simulink model "ES249A_MotAgCorrln"  (R2013b)
settings: Solver=FixedStepDiscrete  SolverMode=SingleTasking  StartTime=0.0  StopTime=1  FixedStep=0.002  RelTol=1e-3
undefined symbols (not defined in the file): FLTINJ_MOTAGCORRLN_MOTAGIDPTSIG, HALFREV_MOTREV_U0P16, MOTAGACORRLNST_CNT_U08, MotAgAMotAgBCorrln, MotAgAMotAgCCorrln, MOTAGBCORRLNST_CNT_U08, MotAgBMotAgCCorrln, MOTAGCCORRLNST_CNT_U08, MOTAGCORRLNERRTHD_MOTREVELEC_U0P16, MOTAGCORRLNNTCFAILSTEP_CNT_U16, MOTAGCORRLNNTCPASSSTEP_CNT_U16, MOTAGMAXSTALLCNTR_CNT_U08, MotAgMeclCorrlnSt, MotAgMeclIdptSig, NtcSts1, sigbuilder_block, SysGlbPrmMotPoleCnt
libraries: simulink x5
(part 1 of 4)
settings Model: Creator=pz79n7  LastModifiedBy=FZG88Y
settings SolverCC: AutoInsertRateTranBlk=on  InsertRTBMode=Always
settings DataIOCC: LimitDataPoints=off  SaveFormat=Structure  ReturnWorkspaceOutputs=on
settings OptimizationCC: BlockReduction=off  InlineParams=on  ZeroExternalMemoryAtStartup=off  ZeroInternalMemoryAtStartup=off  OptimizeModelRefInitCode=on  LifeSpan=1
settings DebuggingCC: SignalInfNanChecking=error  SignalRangeChecking=warning  UnderspecifiedInitializationDetection=Simplified  SolverPrmCheckMsg=error  InheritedTsInSrcMsg=error  DiscreteInheritContinuousMsg=error  SingleTaskRateTransMsg=error  TasksWithSamePriorityMsg=error  SigSpecEnsureSampleTimeMsg=error  CheckMatrixSingularityMsg=error  ParameterUnderflowMsg=error  ParameterPrecisionLossMsg=error  ParameterTunabilityLossMsg=error  FixptConstUnderflowMsg=warning  FixptConstOverflowMsg=warning  VectorMatrixConversionMsg=error  SignalLabelMismatchMsg=error  UnconnectedInputMsg=error  UnconnectedOutputMsg=error  UnconnectedLineMsg=error  SFcnCompatibilityMsg=error  UniqueDataStoreMsg=warning  BusObjectLabelMismatch=error  RootOutportRequireBusObject=error  AssertControl=DisableAll  ModelReferenceIOMsg=error  ModelReferenceVersionMismatchMessage=warning  ModelReferenceIOMismatchMessage=error  ModelReferenceCSMismatchMessage=warning  ModelReferenceDataLoggingMessage=error  StateNameClashWarn=warning  StrictBusMsg=ErrorOnBusTreatedAsVector  NonBusSignalsTreatedAsBus=error  SFUnexpectedBacktrackingDiag=error  SFInvalidInputDataAccessInChartInitDiag=error  SFNoUnconditionalDefaultTransitionDiag=error  SFTransitionOutsideNaturalParentDiag=error  SFUnconditionalTransitionShadowingDiag=error  SFUndirectedBroadcastEventsDiag=error
settings ModelReferenceCC: ModelReferenceNumInstancesAllowed=Single
settings RTWCC: SystemTargetFile=autosar.tlc  GenCodeOnly=on  TemplateMakefile=ert_default_tmf  Description=AUTOSAR  GenerateReport=on  ProcessScript=autosar_make_rtw_hook  LaunchReport=on
settings CodeAppCC: GenerateComments=off  IgnoreCustomStorageClasses=off  CustomSymbolStrType=$N$R$M  CustomSymbolStrBlkIO=$N$M  SimulinkBlockComments=off
settings STFCustomTargetCC: ParMdlRefBuildCompliant=on  CompOptLevelCompliant=on  IncludeMdlTerminateFcn=off  CombineOutputUpdateFcns=on  SuppressErrorStatus=on  ERTFirstTimeCompliant=on  ERTCustomFileBanners=on  SupportNonFinite=off  SupportComplex=off  SupportContinuousTime=off  SupportNonInlinedSFcns=off  MATLABClassNameForMDSCustomization=Simulink.SoftwareTarget.ERTCustomization  AutosarCompliant=on  GRTInterface=off  SystemTargetFile=autosar.tlc
settings ERTTargetCC: CodeReplacementLibrary=ANSI_C  ConcurrentExecutionCompliant=off  IncludeMdlTerminateFcn=off  SuppressErrorStatus=on  SupportNonFinite=off  SupportComplex=off  ModelStepFunctionPrototypeControlCompliant=off  CPPClassGenCompliant=off  AutosarCompliant=on  InlinedParameterPlacement=NonHierarchical  ERTCustomFileTemplate=example_file_process.tlc  EnableUserReplacementTypes=on

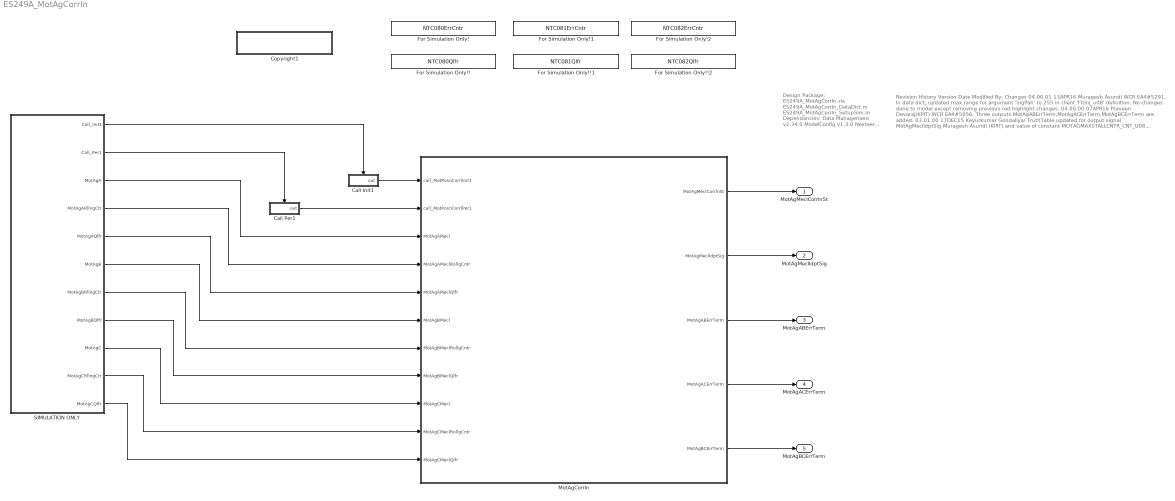
== system ES249A_MotAgCorrln ==
  note: Revision History
      |
      | Version		Date 		Modified By: 		          Changes
      | 04.00.01        13APR16     Muragesh Asundi              WCR EA4#5291, In data dict, updated max range for argument 'SigPah' to 255 in client 'FltInj_u08' definition.
      |                                                                                     No changes done to model except removing previous red highlight changes.
      | 04.00.00        07APR16      Praveen Devaraj(KPIT)    WCR EA4#5056. Three outputs MotAgABErrTerm,MotAgACErrTerm,MotAgBCErrTerm are added.
      | 03.01.00        17DEC15      Keyurkumar Gondaliya/    TruthTable updated for output signal MotAgMeclIdptSig
      |                                             Muragesh Asundi (KPIT)  and value of constant MOTAGMAXSTALLCNTR_CNT_U08
      |                                                                                      changed to 200. Work CR EA4#2808
      | 03.00.00		12NOV15	Erlenbeck		            EA4#2424 anomaly cleanup.  Need to account
      | 										            for rollover in correlation diagnostic.
      | 02.01.01        24AUG15      Muragesh Asundi             Data Dict updated for FltInj_u08 arg2 data type
      |                                                                                      per CR EA4#1391
      | 02.01.00        20AUG15      Muragesh Asundi             Rename FltInj & Bit Set/Not Set Anomaly
      |  										           per CR EA4#1353
      | 02.00.00        07AUG15      Aditya Tikekar                  Fault Injection added for MotAgMeclIdptSig
      |  										           per CR EA4#1161
      | 01.00.00 	02AP15		Kushion			            Initial Release
  note: Design Package:
      | ES249A_MotAgCorrln.slx
      | ES249A_MotAgCorrln_DataDict.m
      | ES249A_MotAgCorrln_SetupSim.m
      |
      | Dependancies:
      |    Data Management v2.34.0
      |    ModelConfig v1.3.0
      |    Nexteer Utilities v4.5.0
      |    Tools v1.10.0
      |
      | Requirement: 2.0
  Call Init1 : Subsystem  TreatAsAtomicUnit=on
  Call Per1 : Subsystem  TreatAsAtomicUnit=on
  Copyright1 : Subsystem  Description=|  mask(Copyright Information){none=on}
      | Copyright info block.                                               
      |                                                                     
      | Place copyright information at the top of every subsystem in design.
      mask prompts: none "No parameters"
      mask help: Place copyright information at the top of every subsystem in design.
      mask Display:
      | NxtrConf = 'Nexteer Confidential';
      | 
      | sys = bdroot; %handle for the current model ("system")
      | first = get_param(sys,'Created');
      | if(isempty(first))
      |     first = datestr(now,'yyyy');
      | else
      |     first = first(end-3:end);  %year is last four digits
      | end
      | 
      | last = get_param(sys,'LastModifiedDate');
      | if isempty(last)
      |     last = datestr(now,'yyyy');
      | else
      |     last = last(end-3:end);
      | end
      | 
      | if strcmp(first,last)
      |     fprintf('%s\nCopyright  %s Nexteer',NxtrConf,first);
      | else
      |     fprintf('%s\n%s%s-%s Nexteer',NxtrConf,char(169),first,last);
      | end
  For Simulation Only! : DataStoreMemory  DataStoreName=NTC080ErrCntr
  For Simulation Only!! : DataStoreMemory  DataStoreName=NTC080Qlfr
  For Simulation Only!!1 : DataStoreMemory  DataStoreName=NTC081Qlfr
  For Simulation Only!!2 : DataStoreMemory  DataStoreName=NTC082Qlfr
  For Simulation Only!1 : DataStoreMemory  DataStoreName=NTC081ErrCntr
  For Simulation Only!2 : DataStoreMemory  DataStoreName=NTC082ErrCntr
  MotAgCorrln : Subsystem
  SIMULATION ONLY : Subsystem
  MotAgMeclCorrlnSt : Outport  RequirementInfo={'linktype_rmi_doors' '0000c47a (/E-STEER Core/SubSystem Specifications/Electrical Actuator/Control Module/FDD Module Requirements/EA4/ES249A_MotAgCorrln DRAFT)' '#ES249A_51' 'true' 'REQ: ES249A_51' '' } %GIDa_d8739ec6_a18f_4415_a443_47ea44f287a3
  MotAgMeclIdptSig : Outport  RequirementInfo={'linktype_rmi_doors' '0000c47a (/E-STEER Core/SubSystem Specifications/Electrical Actuator/Control Module/FDD Module Requirements/EA4/ES249A_MotAgCorrln DRAFT)' '#ES249A_52' 'true' 'REQ: ES249A_52' '' } %GIDa_85b325d8_f6bf_41e3_b16b_50e782c8add7  Port=2
  MotAgABErrTerm : Outport  Port=3
  MotAgACErrTerm : Outport  Port=4
  MotAgBCErrTerm : Outport  Port=5
  wires:
  Call Per1/1(out) -> MotAgCorrln/2(call_MotPosnCorrlPer1)
  MotAgCorrln/1(MotAgMeclCorrlnSt) -> MotAgMeclCorrlnSt/1
  MotAgCorrln/2(MotAgMeclIdptSig) -> MotAgMeclIdptSig/1
  SIMULATION ONLY/3(MotAgA) -> MotAgCorrln/3(MotAgAMecl)
  SIMULATION ONLY/11(MotAgCQlfr) -> MotAgCorrln/11(MotAgCMeclQlfr)
  SIMULATION ONLY/4(MotAgARllngCtr) -> MotAgCorrln/4(MotAgAMeclRollgCntr)
  SIMULATION ONLY/5(MotAgAQlfr) -> MotAgCorrln/5(MotAgAMeclQlfr)
  SIMULATION ONLY/6(MotAgB) -> MotAgCorrln/6(MotAgBMecl)
  SIMULATION ONLY/7(MotAgBRllngCtr) -> MotAgCorrln/7(MotAgBMeclRollgCntr)
  SIMULATION ONLY/8(MotAgBQlfr) -> MotAgCorrln/8(MotAgBMeclQlfr)
  SIMULATION ONLY/9(MotAgC) -> MotAgCorrln/9(MotAgCMecl)
  SIMULATION ONLY/10(MotAgCRllngCtr) -> MotAgCorrln/10(MotAgCMeclRollgCntr)
  Call Init1/1(out) -> MotAgCorrln/1(call_MotPosnCorrlInit1)
  SIMULATION ONLY/1(Call_Init1) -> Call Init1/Enable
  SIMULATION ONLY/2(Call_Per1) -> Call Per1/Enable
  MotAgCorrln/3(MotAgABErrTerm) -> MotAgABErrTerm/1
  MotAgCorrln/4(MotAgACErrTerm) -> MotAgACErrTerm/1
  MotAgCorrln/5(MotAgBCErrTerm) -> MotAgBCErrTerm/1

== system ES249A_MotAgCorrln/Call Init1 ==
  Enable : EnablePort
  Function Call Trigger : simulink/Ports & Subsystems/Function-Call Generator  RequirementInfo={} %GIDa_ff755a2e_49d1_45f7_8591_3ce0ef475338  sample_time=0  numberOfIterations=1
  out : Outport
  wires:
  Function Call Trigger/1 -> out/1

== system ES249A_MotAgCorrln/Call Per1 ==
  Enable : EnablePort
  Function Call Trigger : simulink/Ports & Subsystems/Function-Call Generator  RequirementInfo={} %GIDa_c055ea22_668e_465c_aa17_4b0a8dd99bf7  sample_time=0.002  numberOfIterations=1
  out : Outport
  wires:
  Function Call Trigger/1 -> out/1

== system ES249A_MotAgCorrln/Copyright1 ==

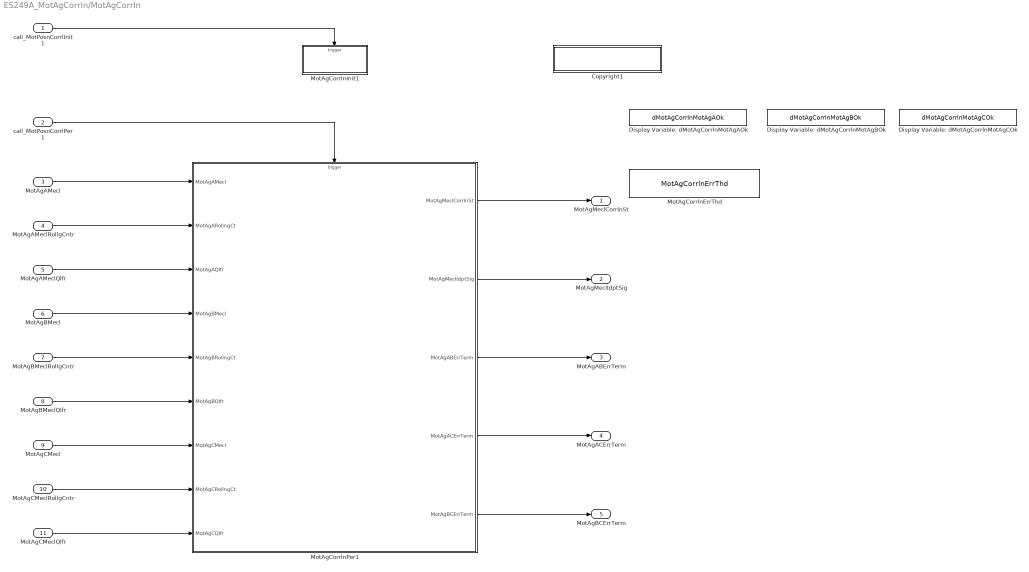
== system ES249A_MotAgCorrln/MotAgCorrln ==
  call_MotPosnCorrlInit1 : Inport  RequirementInfo={} %GIDa_df7b2033_8a98_4878_957d_25acf0131f4b
  call_MotPosnCorrlPer1 : Inport  RequirementInfo={} %GIDa_1551d67e_f818_426a_9cf4_9f4ba82b3f43  Port=2
  MotAgAMecl : Inport  RequirementInfo={'linktype_rmi_doors' '0000c47a (/E-STEER Core/SubSystem Specifications/Electrical Actuator/Control Module/FDD Module Requirements/EA4/ES249A_MotAgCorrln DRAFT)' '#ES249A_48' 'true' 'REQ: ES249A_48' '' } %GIDa_ab802314_3944_43a8_9f34_099947b7f787  Port=3
  MotAgAMeclRollgCntr : Inport  RequirementInfo={'linktype_rmi_doors' '0000c47a (/E-STEER Core/SubSystem Specifications/Electrical Actuator/Control Module/FDD Module Requirements/EA4/ES249A_MotAgCorrln DRAFT)' '#ES249A_49' 'true' 'REQ: ES249A_49' '' } %GIDa_a38bab73_f7bf_4755_8745_3afc46561306  Port=4
  MotAgAMeclQlfr : Inport  RequirementInfo={'linktype_rmi_doors' '0000c47a (/E-STEER Core/SubSystem Specifications/Electrical Actuator/Control Module/FDD Module Requirements/EA4/ES249A_MotAgCorrln DRAFT)' '#ES249A_65' 'true' 'REQ: ES249A_65' '' } %GIDa_033694cf_56a5_4107_96d0_836401cb9721  Port=5
  MotAgBMecl : Inport  RequirementInfo={'linktype_rmi_doors' '0000c47a (/E-STEER Core/SubSystem Specifications/Electrical Actuator/Control Module/FDD Module Requirements/EA4/ES249A_MotAgCorrln DRAFT)' '#ES249A_66' 'true' 'REQ: ES249A_66' '' } %GIDa_ed21c9ba_4edb_4b2f_a77a_49cd20ecbf68  Port=6
  MotAgBMeclRollgCntr : Inport  RequirementInfo={'linktype_rmi_doors' '0000c47a (/E-STEER Core/SubSystem Specifications/Electrical Actuator/Control Module/FDD Module Requirements/EA4/ES249A_MotAgCorrln DRAFT)' '#ES249A_67' 'true' 'REQ: ES249A_67' '' } %GIDa_6e6bb4b4_2d5c_4f1b_b4e7_5884c06a9259  Port=7
  MotAgBMeclQlfr : Inport  RequirementInfo={'linktype_rmi_doors' '0000c47a (/E-STEER Core/SubSystem Specifications/Electrical Actuator/Control Module/FDD Module Requirements/EA4/ES249A_MotAgCorrln DRAFT)' '#ES249A_68' 'true' 'REQ: ES249A_68' '' } %GIDa_842dc15f_0b28_4c0e_80ed_768af48a7cab  Port=8
  MotAgCMecl : Inport  RequirementInfo={'linktype_rmi_doors' '0000c47a (/E-STEER Core/SubSystem Specifications/Electrical Actuator/Control Module/FDD Module Requirements/EA4/ES249A_MotAgCorrln DRAFT)' '#ES249A_69' 'true' 'REQ: ES249A_69' '' } %GIDa_4e69db8b_365e_45b9_94df_b7de55be4fe5  Port=9
  MotAgCMeclRollgCntr : Inport  RequirementInfo={'linktype_rmi_doors' '0000c47a (/E-STEER Core/SubSystem Specifications/Electrical Actuator/Control Module/FDD Module Requirements/EA4/ES249A_MotAgCorrln DRAFT)' '#ES249A_70' 'true' 'REQ: ES249A_70' '' } %GIDa_8619747b_ec91_49fd_b968_535920207abf  Port=10
  MotAgCMeclQlfr : Inport  RequirementInfo={'linktype_rmi_doors' '0000c47a (/E-STEER Core/SubSystem Specifications/Electrical Actuator/Control Module/FDD Module Requirements/EA4/ES249A_MotAgCorrln DRAFT)' '#ES249A_71' 'true' 'REQ: ES249A_71' '' } %GIDa_ccdead46_e253_49ae_a139_b28c04022f0c  Port=11
  Copyright1 : Subsystem  Description=|  RequirementInfo={} %GIDa_dd7bc4e6_4adb_4397_9a47_107977c533a5  mask(Copyright Information){none=on}
      | Copyright info block.                                               
      |                                                                     
      | Place copyright information at the top of every subsystem in design.
      mask prompts: none "No parameters"
      mask help: Place copyright information at the top of every subsystem in design.
      mask Display:
      | NxtrConf = 'Nexteer Confidential';
      | 
      | sys = bdroot; %handle for the current model ("system")
      | first = get_param(sys,'Created');
      | if(isempty(first))
      |     first = datestr(now,'yyyy');
      | else
      |     first = first(end-3:end);  %year is last four digits
      | end
      | 
      | last = get_param(sys,'LastModifiedDate');
      | if isempty(last)
      |     last = datestr(now,'yyyy');
      | else
      |     last = last(end-3:end);
      | end
      | 
      | if strcmp(first,last)
      |     fprintf('%s\nCopyright  %s Nexteer',NxtrConf,first);
      | else
      |     fprintf('%s\n%s%s-%s Nexteer',NxtrConf,char(169),first,last);
      | end
  Display Variable: dMotAgCorrlnMotAgAOk : DataStoreMemory  DataStoreName=dMotAgCorrlnMotAgAOk  StateMustResolveToSignalObject=on
  Display Variable: dMotAgCorrlnMotAgBOk : DataStoreMemory  DataStoreName=dMotAgCorrlnMotAgBOk  StateMustResolveToSignalObject=on
  Display Variable: dMotAgCorrlnMotAgCOk : DataStoreMemory  DataStoreName=dMotAgCorrlnMotAgCOk  StateMustResolveToSignalObject=on
  MotAgCorrlnErrThd : DataStoreMemory  Priority=0  DataStoreName=MotAgCorrlnErrThd  StateMustResolveToSignalObject=on
  MotAgCorrlnInit1 : Subsystem  TreatAsAtomicUnit=on
  MotAgCorrlnPer1 : Subsystem  RequirementInfo={} %GIDa_e8c7526b_9849_4008_8b1a_56f97ffa1c8d  TreatAsAtomicUnit=on
  MotAgMeclCorrlnSt : Outport  RequirementInfo={'linktype_rmi_doors' '0000c47a (/E-STEER Core/SubSystem Specifications/Electrical Actuator/Control Module/FDD Module Requirements/EA4/ES249A_MotAgCorrln DRAFT)' '#ES249A_51' 'true' 'REQ: ES249A_51' '' } %GIDa_ae509c2f_e3de_4035_9028_020cbec86e82
  MotAgMeclIdptSig : Outport  RequirementInfo={'linktype_rmi_doors' '0000c47a (/E-STEER Core/SubSystem Specifications/Electrical Actuator/Control Module/FDD Module Requirements/EA4/ES249A_MotAgCorrln DRAFT)' '#ES249A_52' 'true' 'REQ: ES249A_52' '' } %GIDa_df68f2b0_a0f0_444f_88a1_35645a7edbac  Port=2
  MotAgABErrTerm : Outport  RequirementInfo={'linktype_rmi_doors' '0000c47a (/E-STEER Core/SubSystem Specifications/Electrical Actuator/Control Module/FDD Module Requirements/EA4/ES249A_MotAgCorrln)' '#ES249A_111' 'true' 'REQ: ES249A_111' '' } %GIDa_a7591317_6142_4ab7_82c5_7f600b8953a4  Port=3
  MotAgACErrTerm : Outport  RequirementInfo={'linktype_rmi_doors' '0000c47a (/E-STEER Core/SubSystem Specifications/Electrical Actuator/Control Module/FDD Module Requirements/EA4/ES249A_MotAgCorrln)' '#ES249A_112' 'true' 'REQ: ES249A_112' '' } %GIDa_b9bf6249_4df4_466a_a244_82e9ba0ccbfb  Port=4
  MotAgBCErrTerm : Outport  RequirementInfo={'linktype_rmi_doors' '0000c47a (/E-STEER Core/SubSystem Specifications/Electrical Actuator/Control Module/FDD Module Requirements/EA4/ES249A_MotAgCorrln)' '#ES249A_115' 'true' 'REQ: ES249A_115' '' } %GIDa_2a69805f_47c5_4027_96ea_c2a85e934646  Port=5
  wires:
  call_MotPosnCorrlPer1/1 -> MotAgCorrlnPer1/Trigger
  MotAgCorrlnPer1/2(MotAgMeclIdptSig) -> MotAgMeclIdptSig/1
  MotAgCorrlnPer1/1(MotAgMeclCorrlnSt) -> MotAgMeclCorrlnSt/1
  MotAgAMecl/1 -> MotAgCorrlnPer1/1(MotAgAMecl)
  MotAgAMeclRollgCntr/1 -> MotAgCorrlnPer1/2(MotAgARollngCt)
  MotAgAMeclQlfr/1 -> MotAgCorrlnPer1/3(MotAgAQlfr)
  MotAgBMecl/1 -> MotAgCorrlnPer1/4(MotAgBMecl)
  MotAgBMeclRollgCntr/1 -> MotAgCorrlnPer1/5(MotAgBRollngCt)
  MotAgBMeclQlfr/1 -> MotAgCorrlnPer1/6(MotAgBQlfr)
  MotAgCMecl/1 -> MotAgCorrlnPer1/7(MotAgCMecl)
  MotAgCMeclRollgCntr/1 -> MotAgCorrlnPer1/8(MotAgCRollngCt)
  MotAgCMeclQlfr/1 -> MotAgCorrlnPer1/9(MotAgCQlfr)
  call_MotPosnCorrlInit1/1 -> MotAgCorrlnInit1/Trigger
  MotAgCorrlnPer1/3(MotAgABErrTerm) -> MotAgABErrTerm/1
  MotAgCorrlnPer1/4(MotAgACErrTerm) -> MotAgACErrTerm/1
  MotAgCorrlnPer1/5(MotAgBCErrTerm) -> MotAgBCErrTerm/1

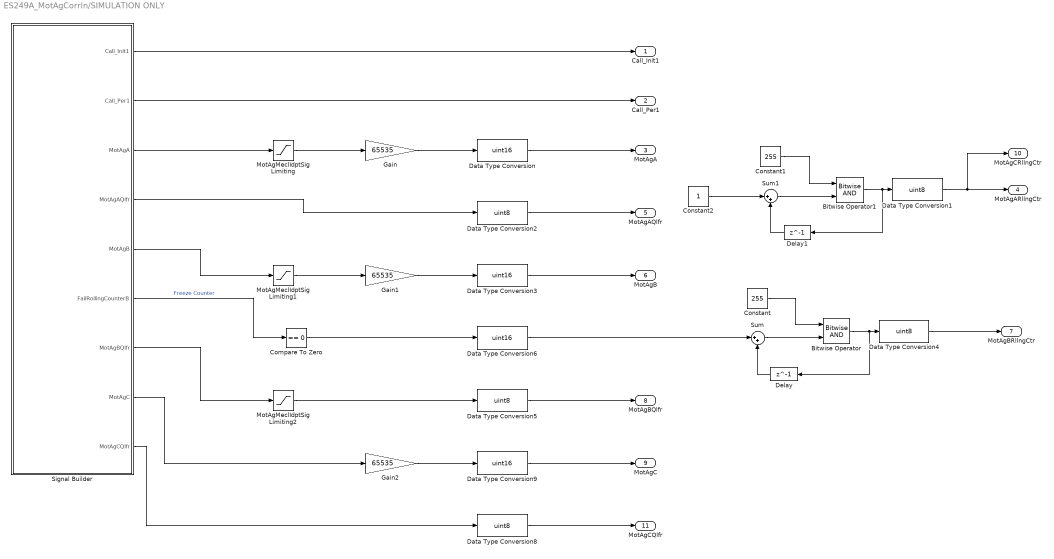
== system ES249A_MotAgCorrln/SIMULATION ONLY ==
  Bitwise Operator : simulink/Logic and Bit Operations/Bitwise Operator  logicop=AND  UseBitMask=off  NumInputPorts=2  BitMask=bin2dec('11011001')  BitMaskRealWorld=Stored Integer
  Bitwise Operator1 : simulink/Logic and Bit Operations/Bitwise Operator  logicop=AND  UseBitMask=off  NumInputPorts=2  BitMask=bin2dec('11011001')  BitMaskRealWorld=Stored Integer
  Compare To Zero : simulink/Logic and Bit Operations/Compare To Zero  relop===  OutDataTypeStr=boolean
  Constant : Constant  Value=255  OutDataTypeStr=uint16
  Constant1 : Constant  Value=255  OutDataTypeStr=uint16
  Constant2 : Constant  OutDataTypeStr=uint16
  Data Type Conversion{,3,6,9} (4 alike) : DataTypeConversion  OutDataTypeStr=uint16
  Data Type Conversion{1..2,4..5,8} (5 alike) : DataTypeConversion  OutDataTypeStr=uint8
  Delay : Delay  DelayLength=1  InitialCondition=0  SampleTime=0.002
  Delay1 : Delay  DelayLength=1  InitialCondition=0  SampleTime=0.002
  Gain : Gain  Gain=65535
  Gain1 : Gain  Gain=65535
  Gain2 : Gain  Gain=65535
  MotAgMeclIdptSig Limiting : Saturate  UpperLimit=1  LowerLimit=0
  MotAgMeclIdptSig Limiting1 : Saturate  UpperLimit=MotAgMeclIdptSig.EngMax  LowerLimit=MotAgMeclIdptSig.EngMin
  MotAgMeclIdptSig Limiting2 : Saturate  UpperLimit=MotAgMeclIdptSig.EngMax  LowerLimit=MotAgMeclIdptSig.EngMin
  Signal Builder : Subsystem  Tag=STV Subsys  LoadFcn=sigbuilder_block('load');  StartFcn=sigbuilder_block('start');  StopFcn=sigbuilder_block('stop');  ClipboardFcn=sigbuilder_block('clipboard');  mask(Sigbuilder block){}
      mask help: Simulink:masks:SigbuilderBlock_MD
      mask init:
      | if ~strcmp(get_param(bdroot(gcbh),'SimulationStatus'),'stopped') tuvar = sigbuilder_block('maskInit'); end
      settings: CopyFcn=sigbuilder_block('copy');  DeleteFcn=sigbuilder_block('delete');  ModelCloseFcn=sigbuilder_block('modelClose');  PreSaveFcn=sigbuilder_block('preSave');  PauseFcn=sigbuilder_block('pause');  ContinueFcn=sigbuilder_block('continue');  NameChangeFcn=sigbuilder_block('namechange');  OpenFcn=sigbuilder_block('open',[5.58621 35.3793 1179.31 576 ]);  CloseFcn=sigbuilder_block('close');
      mask Display: plot(0, 0, 100, 100,[2, 2, 32, 32, 2], [68, 8, 8, 68, 68],[32, 2], [38, 38], [32, 19, 2],[53, 60, 44], [32, 17, 17, 2],[16, 16, 31, 31]);txt = getActiveGroup(gcbh);text(2, 100, txt,'verticalAlignment', 'top');
  Sum : Sum  Inputs=|++
  Sum1 : Sum  Inputs=|++
  Call_Init1 : Outport
  Call_Per1 : Outport  Port=2
  MotAgA : Outport  Port=3
  MotAgARllngCtr : Outport  Port=4
  MotAgAQlfr : Outport  Port=5
  MotAgB : Outport  Port=6
  MotAgBRllngCtr : Outport  Port=7
  MotAgBQlfr : Outport  Port=8
  MotAgC : Outport  Port=9
  MotAgCRllngCtr : Outport  Port=10
  MotAgCQlfr : Outport  Port=11
  wires:
  Gain2/1 -> Data Type Conversion9/1
  Signal Builder/3(MotAgA) -> MotAgMeclIdptSig Limiting/1
  Signal Builder/4(MotAgAQlfr) -> Data Type Conversion2/1
  Signal Builder/5(MotAgB) -> MotAgMeclIdptSig Limiting1/1
  Signal Builder/7(MotAgBQlfr) -> MotAgMeclIdptSig Limiting2/1
  Signal Builder/8(MotAgC) -> Gain2/1
  Signal Builder/9(MotAgCQlfr) -> Data Type Conversion8/1
  Gain/1 -> Data Type Conversion/1
  Gain1/1 -> Data Type Conversion3/1
  Data Type Conversion4/1 -> MotAgBRllngCtr/1
  Data Type Conversion/1 -> MotAgA/1
  Data Type Conversion2/1 -> MotAgAQlfr/1
  Data Type Conversion5/1 -> MotAgBQlfr/1
  Data Type Conversion9/1 -> MotAgC/1
  Data Type Conversion8/1 -> MotAgCQlfr/1
  Signal Builder/6(FailRollingCounterB) -> Compare To Zero/1  "Freeze Counter"
  Data Type Conversion3/1 -> MotAgB/1
  MotAgMeclIdptSig Limiting/1 -> Gain/1
  MotAgMeclIdptSig Limiting1/1 -> Gain1/1
  MotAgMeclIdptSig Limiting2/1 -> Data Type Conversion5/1
  Compare To Zero/1 -> Data Type Conversion6/1
  Data Type Conversion6/1 -> Sum/1
  Delay/1 -> Sum/2
  Constant/1 -> Bitwise Operator/1
  Sum/1 -> Bitwise Operator/2
  Bitwise Operator/1 -> Delay/1, Data Type Conversion4/1
  Delay1/1 -> Sum1/2
  Constant1/1 -> Bitwise Operator1/1
  Sum1/1 -> Bitwise Operator1/2
  Bitwise Operator1/1 -> Data Type Conversion1/1, Delay1/1
  Data Type Conversion1/1 -> MotAgCRllngCtr/1, MotAgARllngCtr/1
  Constant2/1 -> Sum1/1
  Signal Builder/1(Call_Init1) -> Call_Init1/1
  Signal Builder/2(Call_Per1) -> Call_Per1/1

== system ES249A_MotAgCorrln/MotAgCorrln/Copyright1 ==

== system ES249A_MotAgCorrln/MotAgCorrln/MotAgCorrlnInit1 ==
  function : TriggerPort  TriggerType=function-call
  Compute Error Threshold : Subsystem  TreatAsAtomicUnit=on
  Copyright1 : Subsystem  Description=|  RequirementInfo={} %GIDa_76facc10_fa9f_4b93_b759_726016e2f92e  mask(Copyright Information){none=on}
      | Copyright info block.                                               
      |                                                                     
      | Place copyright information at the top of every subsystem in design.
      mask prompts: none "No parameters"
      mask help: Place copyright information at the top of every subsystem in design.
      mask Display:
      | NxtrConf = 'Nexteer Confidential';
      | 
      | sys = bdroot; %handle for the current model ("system")
      | first = get_param(sys,'Created');
      | if(isempty(first))
      |     first = datestr(now,'yyyy');
      | else
      |     first = first(end-3:end);  %year is last four digits
      | end
      | 
      | last = get_param(sys,'LastModifiedDate');
      | if isempty(last)
      |     last = datestr(now,'yyyy');
      | else
      |     last = last(end-3:end);
      | end
      | 
      | if strcmp(first,last)
      |     fprintf('%s\nCopyright  %s Nexteer',NxtrConf,first);
      | else
      |     fprintf('%s\n%s%s-%s Nexteer',NxtrConf,char(169),first,last);
      | end
